simulink subsystem "ideal_rhombic"  (R2022b)
settings: Solver=VariableStepAuto  StartTime=0.0  StopTime=10.0  RelTol=1e-3
undefined symbols (not defined in the file or in its folder): impulse_torque, rhombic_drive
libraries: fl_lib x12, nesl_utility x3
settings Model: Creator=wilde  LastModifiedBy=wilde

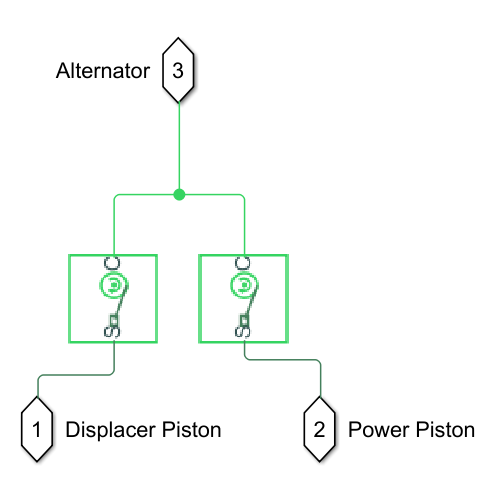
[thumbnail: Simulink's stored preview of the top-level diagram]
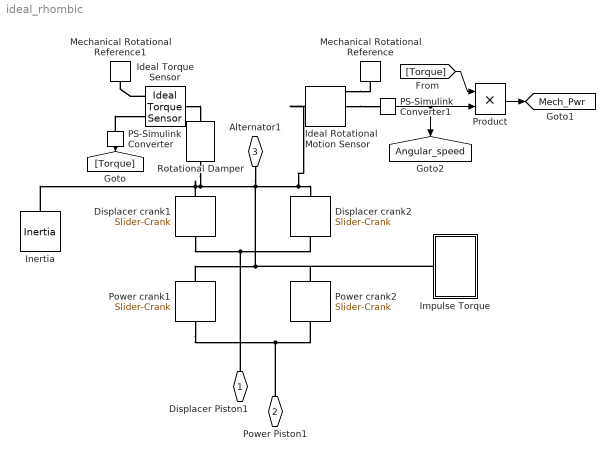
== system ideal_rhombic ==
  Displacer crank1 : fl_lib/Mechanical/Mechanisms/Slider-Crank  crank=rhombic_drive.drive.disp_crank_radius m  rod=rhombic_drive.drive.disp_link_length m  inertia=eps kg*m^2  k=1e7 N/m  b=1e3 N*s/m  theta_specify=on  theta_priority=High  theta=pi / 2 rad  theta_nominal_specify=off  theta_nominal_unit=deg  theta_nominal_value=180  w_specify=on  w_priority=High  w=0 rad/s  w_nominal_specify=off  w_nominal_unit=rad/s  w_nominal_value=1
      settings: InternalSimscapePortConfiguration="{\"Bottom\":[],\"Left\":[{\"id\":\"C\",\"label\":\"C\",\"type\":\"foundation.mechanical.rotational.rotational\"}],\"Right\":[{\"id\":\"S\",\"label\":\"S\",\"type\":\"foundation.mechanical.translational.translational\"}],\"Top\":[]}"
  Displacer crank2 : fl_lib/Mechanical/Mechanisms/Slider-Crank  crank=rhombic_drive.drive.disp_crank_radius m  rod=rhombic_drive.drive.disp_link_length m  inertia=eps kg*m^2  k=1e7 N/m  b=1e3 N*s/m  theta_specify=on  theta_priority=High  theta=pi / 2 rad  theta_nominal_specify=off  theta_nominal_unit=deg  theta_nominal_value=0  w_specify=on  w_priority=High  w=0 rad/s  w_nominal_specify=off  w_nominal_unit=rad/s  w_nominal_value=1
      settings: InternalSimscapePortConfiguration="{\"Bottom\":[],\"Left\":[{\"id\":\"C\",\"label\":\"C\",\"type\":\"foundation.mechanical.rotational.rotational\"}],\"Right\":[{\"id\":\"S\",\"label\":\"S\",\"type\":\"foundation.mechanical.translational.translational\"}],\"Top\":[]}"
  Ideal Rotational Motion Sensor : fl_lib/Mechanical/Mechanical Sensors/Ideal Rotational Motion Sensor  reference=foundation.enum.MeasurementReference.difference  acceleration_port=false  velocity_port=true  position_port=true  wrap_angle=false  offset=0 rad
  Ideal Torque Sensor : fl_lib/Mechanical/Mechanical Sensors/Ideal Torque Sensor
  Impulse Torque : Subsystem  Tag=Impulse Torquw
  Inertia : fl_lib/Mechanical/Rotational Elements/Inertia  inertia=rhombic_drive.geom.crank_inertia kg*m^2  num_ports=foundation.enum.numPorts2.one  w_specify=on  w_priority=High  w=0 rad/s  w_nominal_specify=off  w_nominal_unit=rad/s  w_nominal_value=1  t_specify=off  t_priority=None  t=0 N*m  t_nominal_specify=off  t_nominal_unit=N*m  t_nominal_value=1
  Mechanical Rotational Reference : fl_lib/Mechanical/Rotational Elements/Mechanical Rotational Reference
  Mechanical Rotational Reference1 : fl_lib/Mechanical/Rotational Elements/Mechanical Rotational Reference
  PS-Simulink Converter : nesl_utility/PS-Simulink Converter  PhysicalDomain=network_engine_domain  SubClassName=ps_output  LeftPortType=input  RightPortType=output  PseudoPeriodic=off  Frequencies=[]  VectorFormat=inherit  Unit=inherit  AffineConversion=off
  PS-Simulink Converter1 : nesl_utility/PS-Simulink Converter  PhysicalDomain=network_engine_domain  SubClassName=ps_output  LeftPortType=input  RightPortType=output  PseudoPeriodic=off  Frequencies=[]  VectorFormat=inherit  Unit=inherit  AffineConversion=off
  Power crank1 : fl_lib/Mechanical/Mechanisms/Slider-Crank  crank=rhombic_drive.drive.power_crank_radius m  rod=rhombic_drive.drive.power_link_length m  inertia=eps kg*m^2  k=1e7 N/m  b=1e3 N*s/m  theta_specify=on  theta_priority=High  theta=0 rad  theta_nominal_specify=off  theta_nominal_unit=deg  theta_nominal_value=180  w_specify=off  w_priority=High  w=0 rad/s  w_nominal_specify=off  w_nominal_unit=rad/s  w_nominal_value=1
      settings: InternalSimscapePortConfiguration="{\"Bottom\":[],\"Left\":[{\"id\":\"C\",\"label\":\"C\",\"type\":\"foundation.mechanical.rotational.rotational\"}],\"Right\":[{\"id\":\"S\",\"label\":\"S\",\"type\":\"foundation.mechanical.translational.translational\"}],\"Top\":[]}"
  Power crank2 : fl_lib/Mechanical/Mechanisms/Slider-Crank  crank=rhombic_drive.drive.power_crank_radius m  rod=rhombic_drive.drive.power_link_length m  inertia=eps kg*m^2  k=1e7 N/m  b=1e3 N*s/m  theta_specify=on  theta_priority=High  theta=0 rad  theta_nominal_specify=off  theta_nominal_unit=deg  theta_nominal_value=0  w_specify=off  w_priority=High  w=0 rad/s  w_nominal_specify=off  w_nominal_unit=rad/s  w_nominal_value=1
      settings: InternalSimscapePortConfiguration="{\"Bottom\":[],\"Left\":[{\"id\":\"C\",\"label\":\"C\",\"type\":\"foundation.mechanical.rotational.rotational\"}],\"Right\":[{\"id\":\"S\",\"label\":\"S\",\"type\":\"foundation.mechanical.translational.translational\"}],\"Top\":[]}"
  Product : Product
  Rotational Damper : fl_lib/Mechanical/Rotational Elements/Rotational Damper  D=rhombic_drive.rot_damp N*m*s/rad  w_specify=off  w_priority=None  w=0 rad/s  w_nominal_specify=off  w_nominal_unit=rad/s  w_nominal_value=1  t_specify=off  t_priority=None  t=0 N*m  t_nominal_specify=off  t_nominal_unit=N*m  t_nominal_value=1
  Displacer Piston1 : PMIOPort  Side=Right
  Power Piston1 : PMIOPort  Port=2  Side=Left
  Alternator1 : PMIOPort  Port=3  Side=Left
  tag scope: Angular_speed=global, Mech_Pwr=global
  wires:
  PS-Simulink Converter/1 -> [Torque]
  [Torque] -> Product/1
  PS-Simulink Converter1/1 -> Product/2, [Angular_speed]
  Product/1 -> [Mech_Pwr]
  connections:
  Displacer crank1/RConn1 -- Displacer crank2/RConn1 -- Displacer Piston1/RConn1
  Power Piston1/RConn1 -- Power crank2/RConn1 -- Power crank1/RConn1
  Inertia/LConn1 -- Power crank2/LConn1 -- Impulse Torque/LConn1 -- Power crank1/LConn1 -- Alternator1/RConn1 -- Displacer crank2/LConn1 -- Ideal Rotational Motion Sensor/LConn1 -- Rotational Damper/LConn1 -- Displacer crank1/LConn1
  Ideal Rotational Motion Sensor/RConn1 -- Mechanical Rotational Reference/LConn1
  Ideal Torque Sensor/RConn1 -- Mechanical Rotational Reference1/LConn1
  PS-Simulink Converter/LConn1 -- Ideal Torque Sensor/RConn2
  Ideal Rotational Motion Sensor/RConn2 -- PS-Simulink Converter1/LConn1
  Ideal Torque Sensor/LConn1 -- Rotational Damper/RConn1

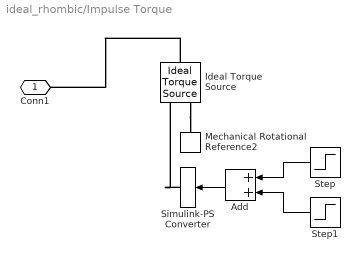
== system ideal_rhombic/Impulse Torque ==
  Add : Sum
  Ideal Torque Source : fl_lib/Mechanical/Mechanical Sources/Ideal Torque Source
  Mechanical Rotational Reference2 : fl_lib/Mechanical/Rotational Elements/Mechanical Rotational Reference
  Simulink-PS Converter : nesl_utility/Simulink-PS Converter  PhysicalDomain=network_engine_domain  SubClassName=ps_input  LeftPortType=input  RightPortType=output  PseudoPeriodic=off  Frequencies=[]  NoiseDistribution=none  NoiseParameters=[]  Unit=N*m  AffineConversion=off  FilteringAndDerivatives=filter  SimscapeFilterOrder=1  InputFilterTimeConstant=0.001  UdotUserProvided=0
  Step : Step  Time=impulse_torque.t_end  Before=impulse_torque.torque  After=0  SampleTime=0
  Step1 : Step  Time=impulse_torque.t_start  Before=- impulse_torque.torque  After=0  SampleTime=0
  Conn1 : PMIOPort  Side=Left
  wires:
  Add/1 -> Simulink-PS Converter/1
  Step/1 -> Add/1
  Step1/1 -> Add/2
  connections:
  Ideal Torque Source/LConn1 -- Conn1/RConn1
  Simulink-PS Converter/RConn1 -- Ideal Torque Source/RConn1
  Ideal Torque Source/RConn2 -- Mechanical Rotational Reference2/LConn1
